simulink model "gm_hdlcoder_led_blinking_interface"  (R2019a)
settings: Solver=FixedStepDiscrete  StartTime=0.0  StopTime=inf  RelTol=1e-3  EnableMultiTasking=on
InitFcn:
  | Ts = 1e-3;
undefined symbols (not defined in the file): AXI4, Lite
libraries: axiinterfacelib x3, simulink x2
settings Model: SimulationMode=external  Creator=The MathWorks, Inc.  LastModifiedBy=rbhar
settings SolverCC: ConcurrentTasks=on  PositivePriorityOrder=on
settings DataIOCC: LimitDataPoints=on  SaveFormat=Array  SaveOutput=off  SignalLogging=off  SaveTime=off  ReturnWorkspaceOutputs=off
settings OptimizationCC: BlockReduction=off  ConditionallyExecuteInputs=off  EnhancedBackFolding=on  PassReuseOutputArgsAs=Individual arguments  ExpressionDepthLimit=2147483647  MaxStackSize=64  OptimizeBlockOrder=speed  DifferentSizesBufferReuse=on  OptimizationCustomize=off
settings DebuggingCC: AlgebraicLoopMsg=error  UnderspecifiedInitializationDetection=Classic  MergeDetectMultiDrivingBlocksExec=none  SolverPrmCheckMsg=warning  SingleTaskRateTransMsg=error  ParameterPrecisionLossMsg=none  ParameterTunabilityLossMsg=error  StateNameClashWarn=warning  SFUnexpectedBacktrackingDiag=warning  SFNoUnconditionalDefaultTransitionDiag=warning  SFExecutionAtInitializationDiag=none  ArithmeticOperatorsInVariantConditions=warning
settings HardwareCC: ProdBitPerPointer=32  ProdBitPerSizeT=32  ProdBitPerPtrDiffT=32  ProdLargestAtomicInteger=Long  ProdLargestAtomicFloat=Double  ProdWordSize=32  ProdHWDeviceType=ARM Compatible->ARM Cortex  TargetEndianess=LittleEndian
settings ModelReferenceCC: PropagateSignalLabelsOutOfModel=off
settings SFSimCC: SimUseLocalCustomCode=off  MATLABDynamicMemAlloc=off
settings RTWCC: SystemTargetFile=ert.tlc  HardwareBoard=ZedBoard  TLCOptions="-aInlineSetEventsForThisBaseRateFcn=TLC_FALSE -aSuppressMultiTaskScheduler=TLC_FALSE  -aRateBasedStepFcn=0"  TemplateMakefile=ert_default_tmf  GenerateReport=on  RTWUseLocalCustomCode=off  Toolchain=Linaro AArch32 Linux v6.3.1  IncludeHyperlinkInReport=on  LaunchReport=on  GenerateTraceInfo=on  GenerateTraceReport=on  GenerateTraceReportSl=on  GenerateTraceReportSf=on  GenerateTraceReportEml=on
settings CodeAppCC: ForceParamTrailComments=on  IgnoreCustomStorageClasses=off  OperatorAnnotations=on  SimulinkDataObjDesc=on  SFDataObjDesc=on  InsertBlockDesc=on
settings ConfigComp: CovMetricSettings=dw  CovHtmlReporting=on  CovSaveCumulativeToWorkspaceVar=on  CovSaveSingleToWorkspaceVar=on  CovExternalEMLEnable=off

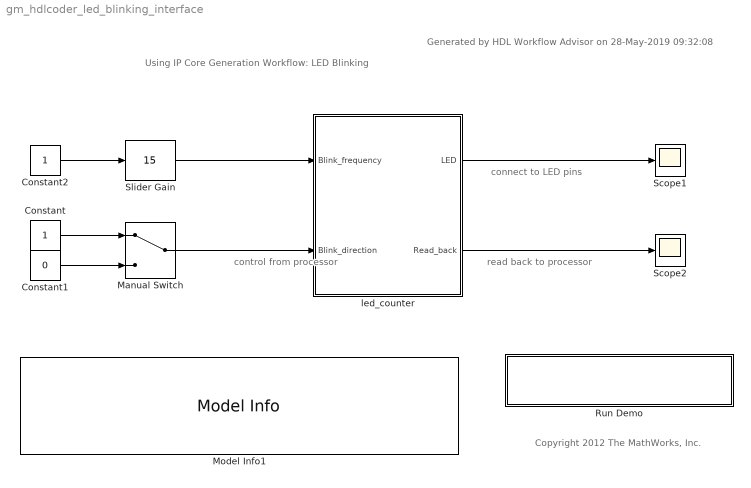
== system gm_hdlcoder_led_blinking_interface ==
  note: read back to
      | processor
  note: connect to
      | LED pins
  note: control from
      | processor
  note: Using IP Core Generation Workflow: LED Blinking
  note: Copyright 2012 The MathWorks, Inc.
  note: Generated by HDL Workflow Advisor on 28-May-2019 09:32:08
  Constant : Constant  OutDataTypeStr=boolean  SampleTime=Ts
  Constant1 : Constant  Value=0  OutDataTypeStr=boolean  SampleTime=Ts
  Constant2 : Constant  OutDataTypeStr=fixdt(0, 4, 0)  SampleTime=Ts
  Manual Switch : ManualSwitch
  Model Info1 : simulink/Model-Wide Utilities/Model Info  Frame=on  DisplayStringWithTags=|  HorizontalTextAlignment=Left  LeftAlignmentValue=0.02
      | This example shows how to use HDL Workflow Advisor to 
      | generate a custom IP core which blink LEDs on FPGA board.
      | 
      | In MATLAB, type the following:
      |   hdladvisor('hdlcoder_led_blinking/led_counter')
  Run Demo : Subsystem
      settings: OpenFcn=hdladvisor([bdroot, '/led_counter'])
      mask Display: disp('Launch HDL Workflow Advisor')
  Scope1 : Scope
  Scope2 : Scope
  Slider Gain : simulink/Math Operations/Slider Gain  gain=15  low=0  high=15
  led_counter : Subsystem  TreatAsAtomicUnit=on  mask(AXI4-Lite/AXI4 Interface){}
      mask help:
      | This is an automatically generated subsystem block.
      | This contains the AXI interface blocks that communicate with the led_count_ip IPCore generated from hdlcoder_led_blinking/led_counter subsystem.
      mask Display: disp(sprintf('Xilinx Zynq \nAXI Interface'));
  wires:
  led_counter/1(LED) -> Scope1/1
  led_counter/2(Read_back) -> Scope2/1
  Slider Gain/1 -> led_counter/1(Blink_frequency)
  Constant2/1 -> Slider Gain/1
  Manual Switch/1 -> led_counter/2(Blink_direction)
  Constant1/1 -> Manual Switch/2
  Constant/1 -> Manual Switch/1

== system gm_hdlcoder_led_blinking_interface/Run Demo ==

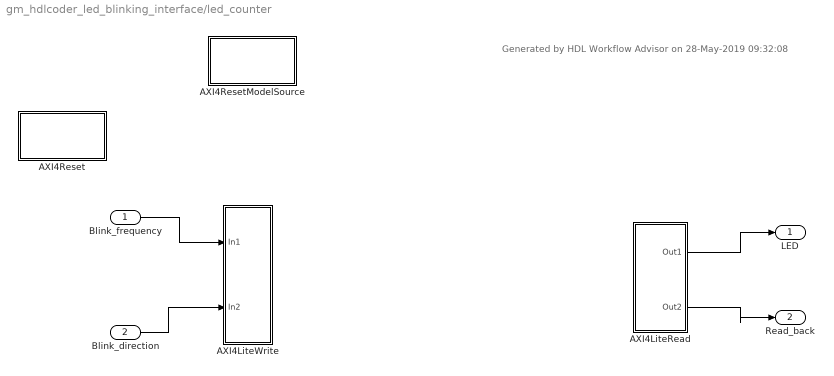
== system gm_hdlcoder_led_blinking_interface/led_counter ==
  note: Generated by HDL Workflow Advisor on 28-May-2019 09:32:08
  Blink_frequency : Inport  OutDataTypeStr=fixdt(0, 4, 0)
  Blink_direction : Inport  Port=2  OutDataTypeStr=boolean
  AXI4LiteRead : Subsystem  Priority=10
  AXI4LiteWrite : Subsystem  Priority=1
  AXI4Reset : Subsystem  mask(System Start){ShowInLibBrowser=0}
      mask prompts: ShowInLibBrowser "Simulink:masks:CustCodeMaskParam1_MP"
      settings: CopyFcn=cccopyfcn(gcb)  OpenFcn=ccopenfcn('System Start Function')
      mask Help: eval('feval(''rtwprivate'',''rtwhelpview'',''rtw_sys_start_block'')');
      mask Display: disp('System\nStart');
  AXI4ResetModelSource : Subsystem  mask(Model Source){ShowInLibBrowser=0}
      mask prompts: ShowInLibBrowser "Simulink:masks:CustCodeMaskParam1_MP"
      settings: CopyFcn=cccopyfcn(gcb)  OpenFcn=ccopenfcn('Model Source')
      mask Help: eval('feval(''rtwprivate'',''rtwhelpview'',''rtw_model_source_block'')');
      mask Display: disp('Model\nSource');
  LED : Outport
  Read_back : Outport  Port=2
  wires:
  Blink_frequency/1 -> AXI4LiteWrite/1(In1)
  Blink_direction/1 -> AXI4LiteWrite/2(In2)
  AXI4LiteRead/1(Out1) -> LED/1
  AXI4LiteRead/2(Out2) -> Read_back/1

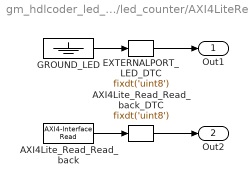
== system gm_hdlcoder_led_blinking_interface/led_counter/AXI4LiteRead ==
  AXI4Lite_Read_Read_back : axiinterfacelib/AXI4-Interface Read  Priority=3  AXIInterfaceType=AXI4-Lite  DeviceName=/dev/mwipcore  RegisterOffset=hex2dec('108')  DataLength=1  DataType=uint32  SampleTime=-1  blockPlatform=ZYNQ  SimulateUsing=Interpreted Execution
      settings: SourceProductName=Embedded Coder Support Package for Xilinx Zynq Platform  SourceProductBaseCode=ECZYNQ7000
  AXI4Lite_Read_Read_back_DTC : DataTypeConversion  OutDataTypeStr=fixdt('uint8')  ConvertRealWorld=Stored Integer (SI)
  EXTERNALPORT_LED_DTC : DataTypeConversion  OutDataTypeStr=fixdt('uint8')
  GROUND_LED : Ground
  Out1 : Outport
  Out2 : Outport  Port=2
  wires:
  AXI4Lite_Read_Read_back/1 -> AXI4Lite_Read_Read_back_DTC/1
  EXTERNALPORT_LED_DTC/1 -> Out1/1
  AXI4Lite_Read_Read_back_DTC/1 -> Out2/1
  GROUND_LED/1 -> EXTERNALPORT_LED_DTC/1

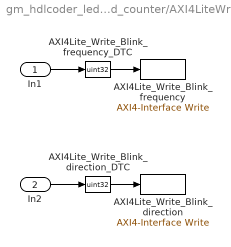
== system gm_hdlcoder_led_blinking_interface/led_counter/AXI4LiteWrite ==
  In1 : Inport
  In2 : Inport  Port=2
  AXI4Lite_Write_Blink_direction : axiinterfacelib/AXI4-Interface Write  Priority=2  AXIInterfaceType=AXI4-Lite  DeviceName=/dev/mwipcore  RegisterOffset=hex2dec('104')  blockPlatform=ZYNQ  SimulateUsing=Interpreted execution
      settings: SourceProductName=Embedded Coder Support Package for Xilinx Zynq Platform  SourceProductBaseCode=ECZYNQ7000
  AXI4Lite_Write_Blink_direction_DTC : DataTypeConversion  OutDataTypeStr=uint32  ConvertRealWorld=Stored Integer (SI)
  AXI4Lite_Write_Blink_frequency : axiinterfacelib/AXI4-Interface Write  Priority=1  AXIInterfaceType=AXI4-Lite  DeviceName=/dev/mwipcore  RegisterOffset=hex2dec('100')  blockPlatform=ZYNQ  SimulateUsing=Interpreted execution
      settings: SourceProductName=Embedded Coder Support Package for Xilinx Zynq Platform  SourceProductBaseCode=ECZYNQ7000
  AXI4Lite_Write_Blink_frequency_DTC : DataTypeConversion  OutDataTypeStr=uint32  ConvertRealWorld=Stored Integer (SI)
  wires:
  AXI4Lite_Write_Blink_direction_DTC/1 -> AXI4Lite_Write_Blink_direction/1
  AXI4Lite_Write_Blink_frequency_DTC/1 -> AXI4Lite_Write_Blink_frequency/1
  In2/1 -> AXI4Lite_Write_Blink_direction_DTC/1
  In1/1 -> AXI4Lite_Write_Blink_frequency_DTC/1

== system gm_hdlcoder_led_blinking_interface/led_counter/AXI4Reset ==

== system gm_hdlcoder_led_blinking_interface/led_counter/AXI4ResetModelSource ==
